simulink model "VDSUV"  (R2020b)
settings: Solver=VariableStepAuto  StartTime=0.0  StopTime=4  RelTol=1e-3
values from neighbouring files (symbols this model uses):
  AirDensity = 1.2256    [VDSUVSimlink.m]    (also in VDSafari.m)
  AirDragCoefficient = 0.45    [VDSUVSimlink.m]    (also in VDSafari.m)
  AllowedFrontLoad = 500 * g    (= 4900)    [VDSUVSimlink.m]    (also in VDSafari.m)
  CarWeight = KerbWeight + DriverWeight    (= 1745)    [VDSUVSimlink.m]    (also in VDSafari.m)
  CoefficientOfFriction = 0.9    [VDSUVSimlink.m]    (also in VDSafari.m)
  CoefficientOfRollingResistance = 0.035    [VDSUVSimlink.m]    (also in VDSafari.m)
  dt = 0.05    [VDSUVSimlink.m]    (also in VDSafari.m)
  Equation = polyfit(EngineRadPs,EngineTorque,2)    [VDSUVSimlink.m]    (also in VDSafari.m)
  FinalDrive = 3.75    [VDSUVSimlink.m]    (also in VDSafari.m)
  FrontalArea = 3.138    [VDSUVSimlink.m]    (also in VDSafari.m)
  FrontWeight = 0.64    [VDSUVSimlink.m]    (also in VDSafari.m)
  FrontWheelRadius = 0.369    [VDSUVSimlink.m]    (also in VDSafari.m)
  g = 9.8    [VDSUVSimlink.m]    (also in VDSafari.m)
  Gears = [1 3.96 ; 2 2.210 ; 3 1.422 ; 4 1 ; 5 0.779 ; 6 0.710]    [VDSUVSimlink.m]    (also in VDSafari.m)
  Height = 0.800    (= 0.8)    [VDSUVSimlink.m]    (also in VDSafari.m)
  MaximumEngineRPM = 3600    [VDSUVSimlink.m]    (also in VDSafari.m)
  MinimumEngineRPM = 1200    [VDSUVSimlink.m]    (also in VDSafari.m)
  Wheelbase = 2.741    [VDSUVSimlink.m]    (also in VDSafari.m)
libraries: simulink x1
settings Model: Creator=dinesh  LastModifiedBy=dinesh
settings DebuggingCC: UnderSpecifiedDimensionMsg=warning

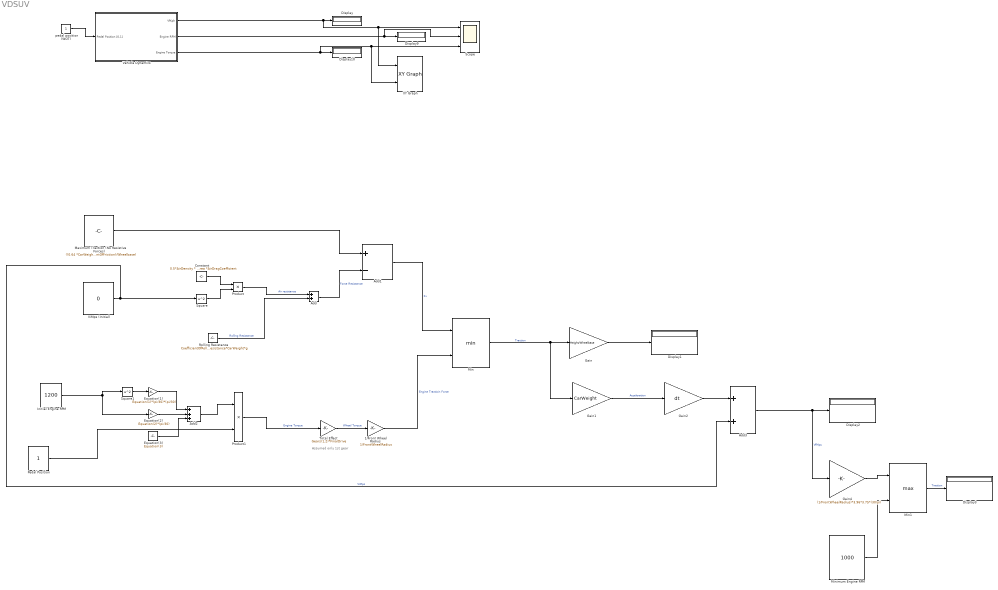
== system VDSUV ==
  note: Assumed only 1st gear
  1/Front Wheel Radius : Gain  Gain=1/FrontWheelRadius
  Add : Sum
  Add1 : Sum  Inputs=+-
  Add2 : Sum  Inputs=+++
  Add3 : Sum
  Constant : Constant  Value=0.5*AirDensity * FrontalArea *AirDragCoefficient
  Display{,1..3,9..10} (6 alike) : Display
  Equation(1) : Gain  Gain=Equation(1)*(pi/30)*(pi/30)
  Equation(2) : Gain  Gain=Equation(2)*(pi/30)
  Equation(3) : Constant  Value=Equation(3)
  Gain : Gain  Gain=Height/Wheelbase
  Gain1 : Gain  Gain=CarWeight
  Gain2 : Gain  Gain=dt
  Gain4 : Gain  Gain=(1/FrontWheelRadius)*3.96*3.75*(30/pi)
  Initial Engine RPM : Constant  Value=1200
  Maximum Traction (No Resistive Forces) : Constant  Value=((0.64 *CarWeight*g*CoefficientOfFriction))/(1+(Height*CoefficientOfFriction)/Wheelbase)
  Min : MinMax  Inputs=2
  Min1 : MinMax  Function=max  Inputs=2
  Minimum Engine RPM : Constant  Value=1000
  Pedal Position : Constant
  Product : Product
  Product1 : Product
  Rolling Resistance : Constant  Value=CoefficientOfRollingResistance*CarWeight*g
  Scope : Scope  NumInputPorts=3
  Square : Math  Operator=square  SaturateOnIntegerOverflow=on
  Square1 : Math  Operator=square  SaturateOnIntegerOverflow=on
  Total Effect : Gain  Gain=Gears(1,2)*FinalDrive
  Vehicle Dynamics : Subsystem
  ViMps (Initial) : Constant  Value=0
  XY Graph : simulink/Sinks/XY Graph  xmin=0  xmax=200  ymin=0  ymax=400  st=dt
  pedal position (WOT) : Constant
  wires:
  pedal position (WOT)/1 -> Vehicle Dynamics/1(Pedal Position [0,1])
  Vehicle Dynamics/1(VfKph) -> XY Graph/1, Scope/1, Display/1
  Vehicle Dynamics/2(Engine RPM) -> Scope/2, Display9/1
  Vehicle Dynamics/3(Engine Torque) -> Scope/3, XY Graph/2, Display10/1
  Add/1 -> Add1/2  "Force Resistance"
  Product/1 -> Add/1  "Air resistance"
  Rolling Resistance/1 -> Add/2  "Rolling Resistance"
  Constant/1 -> Product/1
  Square/1 -> Product/2
  ViMps (Initial)/1 -> Add3/2, Square/1  "ViMps"
  Maximum Traction (No Resistive Forces)/1 -> Add1/1
  1/Front Wheel Radius/1 -> Min/2  "Engine Tractioin Force"
  Product1/1 -> Total Effect/1  "Engine Torque"
  Equation(1)/1 -> Add2/1
  Pedal Position/1 -> Product1/2
  Equation(2)/1 -> Add2/2
  Total Effect/1 -> 1/Front Wheel Radius/1  "Wheel Torque"
  Square1/1 -> Equation(1)/1
  Add2/1 -> Product1/1
  Initial Engine RPM/1 -> Equation(2)/1, Square1/1
  Equation(3)/1 -> Add2/3
  Add1/1 -> Min/1  "Fx"
  Min/1 -> Gain1/1, Gain/1  "Traction"
  Gain/1 -> Display1/1
  Gain1/1 -> Gain2/1  "Acceleration"
  Gain2/1 -> Add3/1
  Add3/1 -> Gain4/1, Display2/1  "VfMps"
  Gain4/1 -> Min1/1
  Minimum Engine RPM/1 -> Min1/2
  Min1/1 -> Display3/1  "Traction"

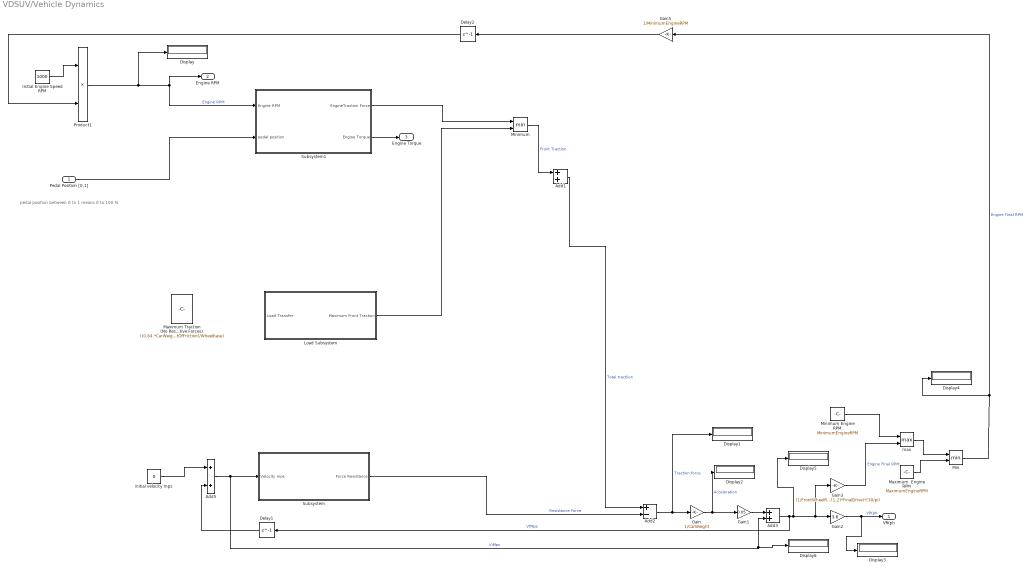
== system VDSUV/Vehicle Dynamics ==
  note: pedal position between 0 to 1 means 0 to 100 %
  Pedal Position [0,1] : Inport
  Add1 : Sum
  Add2 : Sum  Inputs=+-
  Add3 : Sum
  Add5 : Sum
  Delay1 : Delay  DelayLength=1  InitialCondition=0  SampleTime=0.05
  Delay2 : Delay  DelayLength=1  InitialCondition=1  SampleTime=0.05
  Display{,1..6} (7 alike) : Display
  Gain : Gain  Gain=1/CarWeight
  Gain1 : Gain  Gain=0.05
  Gain2 : Gain  Gain=3.6
  Gain3 : Gain  Gain=(1/FrontWheelRadius)*(Gears(1,2)*FinalDrive)*(30/pi)
  Gain5 : Gain  Gain=1/MinimumEngineRPM
  Initial Engine Speed RPM : Constant  Value=1000
  Load Subsystem : Subsystem
  Maximum  Engine RPM : Constant  Value=MaximumEngineRPM
  Maximum Traction (No Resistive Forces) : Constant  Value=((0.64 *CarWeight*g*CoefficientOfFriction))/(1+(Height*CoefficientOfFriction)/Wheelbase)
  Min : MinMax  Inputs=2
  Minimum : MinMax  Inputs=2
  Minimum Engine RPM : Constant  Value=MinimumEngineRPM
  Product1 : Product
  Subsystem : Subsystem
  Subsystem1 : Subsystem
  initial velocity mps : Constant  Value=0
  max : MinMax  Function=max  Inputs=2
  VfKph : Outport
  Engine RPM : Outport  Port=2
  Engine Torque : Outport  Port=3
  wires:
  Load Subsystem/1(Maximum Front Traction) -> Minimum/2
  Minimum/1 -> Add1/1  "Front Traction"
  Subsystem/1(Force Resistance) -> Add2/2  "Resistance Force"
  Add1/1 -> Add2/1  "Total tractiion"
  Add2/1 -> Display1/1, Gain/1  "Traction force"
  Gain/1 -> Display2/1, Gain1/1  "Acceleration"
  Gain1/1 -> Add3/1
  Gain2/1 -> Display3/1, VfKph/1  "VfKph"
  Add3/1 -> Delay1/1, Display5/1, Gain3/1, Gain2/1  "VfMps"
  Gain3/1 -> max/2  "Engine Final RPM"
  Minimum Engine RPM/1 -> max/1
  initial velocity mps/1 -> Add5/1
  Add5/1 -> Display6/1, Add3/2, Subsystem/1(Velocity mps)  "ViMps"
  Delay1/1 -> Add5/2
  Initial Engine Speed RPM/1 -> Product1/1
  Delay2/1 -> Product1/2
  Gain5/1 -> Delay2/1
  max/1 -> Min/1
  Maximum  Engine RPM/1 -> Min/2
  Min/1 -> Display4/1, Gain5/1  "Engine Final RPM"
  Product1/1 -> Display/1, Engine RPM/1, Subsystem1/1(Engine RPM)  "Engine RPM"
  Pedal Position [0,1]/1 -> Subsystem1/2(pedal position)
  Subsystem1/1(EngineTraction Force) -> Minimum/1
  Subsystem1/2(Engine Torque) -> Engine Torque/1

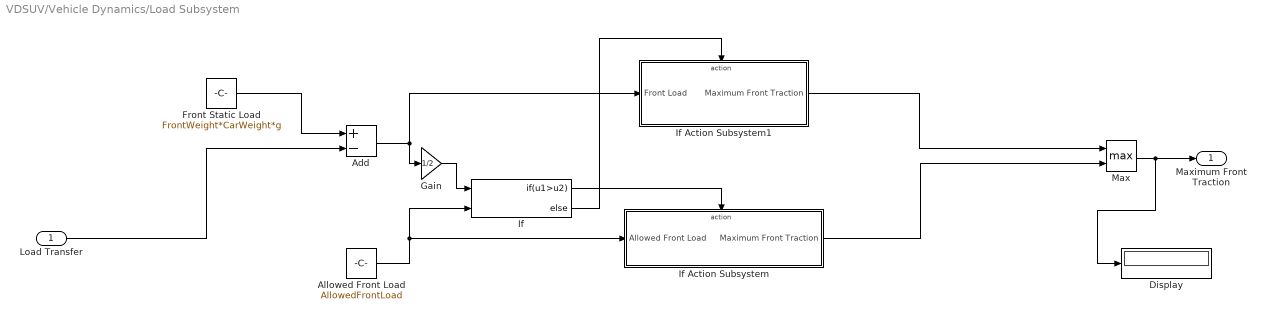
== system VDSUV/Vehicle Dynamics/Load Subsystem ==
  Load Transfer : Inport
  Add : Sum  Inputs=+-
  Allowed Front Load : Constant  Value=AllowedFrontLoad
  Display : Display
  Front Static Load : Constant  Value=FrontWeight*CarWeight*g
  Gain : Gain  Gain=1/2
  If : If  NumInputs=2  IfExpression=u1>u2
  If Action Subsystem : Subsystem  TreatAsAtomicUnit=on
  If Action Subsystem1 : Subsystem  TreatAsAtomicUnit=on
  Max : MinMax  Function=max  Inputs=2
  Maximum Front Traction : Outport
  wires:
  Load Transfer/1 -> Add/2
  Front Static Load/1 -> Add/1
  Add/1 -> Gain/1, If Action Subsystem1/1(Front Load)
  Allowed Front Load/1 -> If/2, If Action Subsystem/1(Allowed Front Load)
  If/1 -> If Action Subsystem/Action
  If/2 -> If Action Subsystem1/Action
  Gain/1 -> If/1
  If Action Subsystem/1(Maximum Front Traction) -> Max/2
  If Action Subsystem1/1(Maximum Front Traction) -> Max/1
  Max/1 -> Display/1, Maximum Front Traction/1

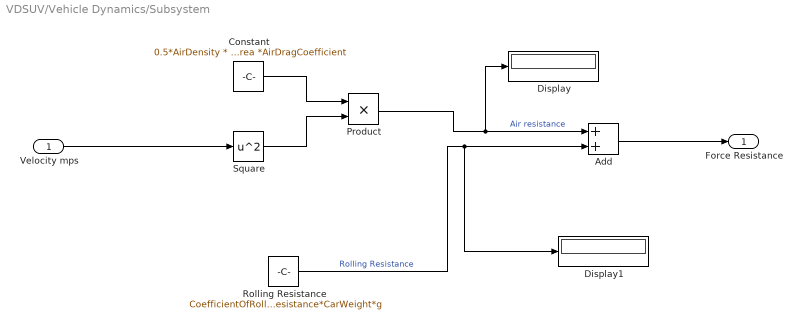
== system VDSUV/Vehicle Dynamics/Subsystem ==
  Velocity mps : Inport
  Add : Sum
  Constant : Constant  Value=0.5*AirDensity * FrontalArea *AirDragCoefficient
  Display : Display
  Display1 : Display
  Product : Product
  Rolling Resistance : Constant  Value=CoefficientOfRollingResistance*CarWeight*g
  Square : Math  Operator=square  SaturateOnIntegerOverflow=on
  Force Resistance : Outport
  wires:
  Velocity mps/1 -> Square/1
  Constant/1 -> Product/1
  Square/1 -> Product/2
  Product/1 -> Display/1, Add/1  "Air resistance"
  Rolling Resistance/1 -> Display1/1, Add/2  "Rolling Resistance"
  Add/1 -> Force Resistance/1

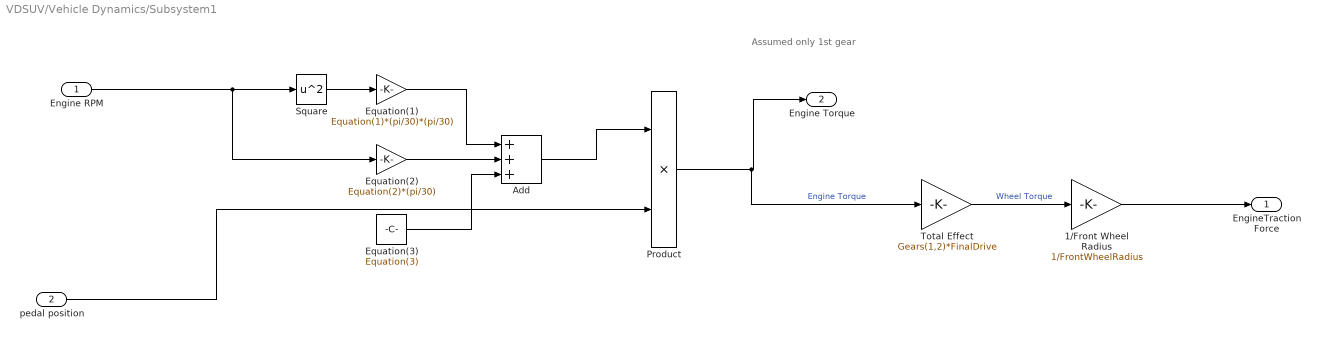
== system VDSUV/Vehicle Dynamics/Subsystem1 ==
  note: Assumed only 1st gear
  Engine RPM : Inport
  pedal position : Inport  Port=2
  1/Front Wheel Radius : Gain  Gain=1/FrontWheelRadius
  Add : Sum  Inputs=+++
  Equation(1) : Gain  Gain=Equation(1)*(pi/30)*(pi/30)
  Equation(2) : Gain  Gain=Equation(2)*(pi/30)
  Equation(3) : Constant  Value=Equation(3)
  Product : Product
  Square : Math  Operator=square  SaturateOnIntegerOverflow=on
  Total Effect : Gain  Gain=Gears(1,2)*FinalDrive
  EngineTraction Force : Outport
  Engine Torque : Outport  Port=2
  wires:
  Add/1 -> Product/1
  Equation(1)/1 -> Add/1
  Equation(3)/1 -> Add/3
  Engine RPM/1 -> Equation(2)/1, Square/1
  Square/1 -> Equation(1)/1
  pedal position/1 -> Product/2
  Total Effect/1 -> 1/Front Wheel Radius/1  "Wheel Torque"
  Equation(2)/1 -> Add/2
  Product/1 -> Total Effect/1, Engine Torque/1  "Engine Torque"
  1/Front Wheel Radius/1 -> EngineTraction Force/1

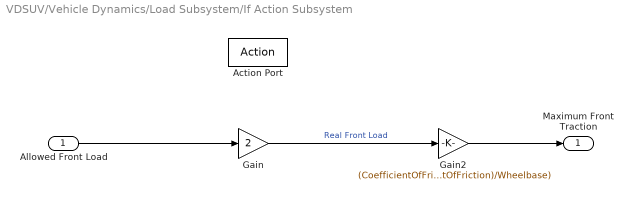
== system VDSUV/Vehicle Dynamics/Load Subsystem/If Action Subsystem ==
  Allowed Front Load : Inport
  Action Port : ActionPort  ActionPortLabel=if(u1>u2)
  Gain : Gain  Gain=2
  Gain2 : Gain  Gain=(CoefficientOfFriction)/(1+(Height*CoefficientOfFriction)/Wheelbase)
  Maximum Front Traction : Outport
  wires:
  Allowed Front Load/1 -> Gain/1
  Gain/1 -> Gain2/1  "Real Front Load"
  Gain2/1 -> Maximum Front Traction/1

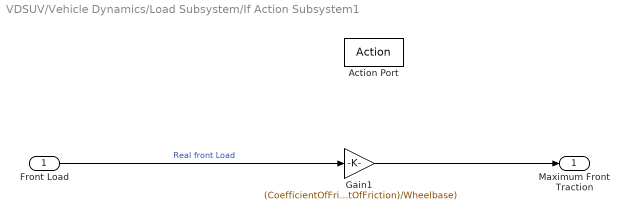
== system VDSUV/Vehicle Dynamics/Load Subsystem/If Action Subsystem1 ==
  Front Load : Inport
  Action Port : ActionPort  ActionPortLabel=else
  Gain1 : Gain  Gain=(CoefficientOfFriction)/(1+(Height*CoefficientOfFriction)/Wheelbase)
  Maximum Front Traction : Outport
  wires:
  Front Load/1 -> Gain1/1  "Real front Load"
  Gain1/1 -> Maximum Front Traction/1
